simulink model "controller"  (R2016b)
settings: Solver=VariableStepAuto  StartTime=0.0  StopTime=10.0  RelTol=1e-3
undefined symbols (not defined in the file): D9, MaxSpeed, PTD5
libraries: simulink x7, frdmkl25zlib x2, slrtlib x2
settings Model: Creator=VasutornSIRIYAKORN  LastModifiedBy=VasutornSIRIYAKORN

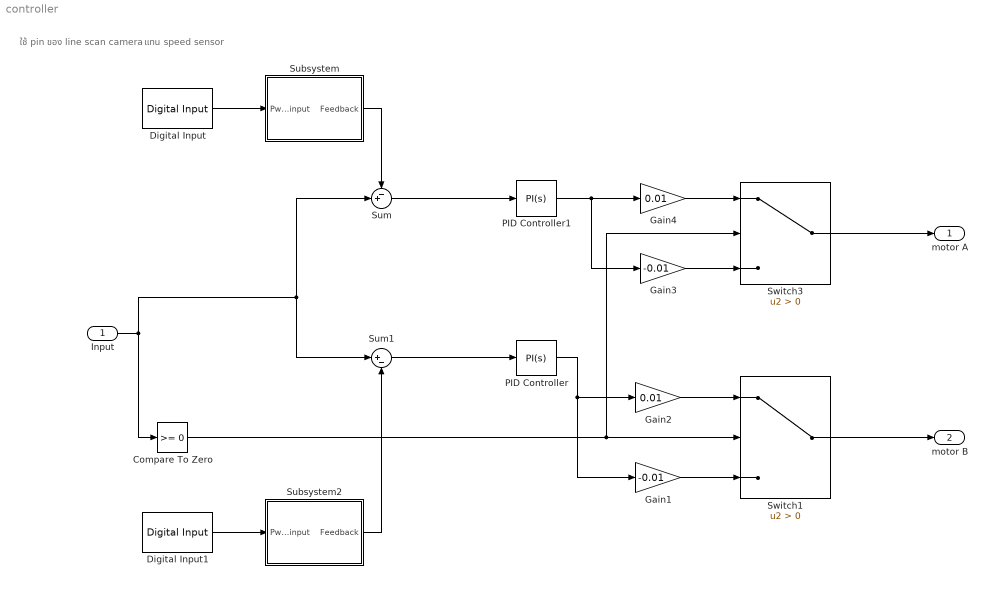
== system controller ==
  note: ใช้ pin ของ line scan camera แทน speed sensor
  "Input " : Inport
  Compare To Zero : simulink/Logic and Bit Operations/Compare To Zero  relop=>=  OutDataTypeStr=boolean
  Digital Input : frdmkl25zlib/Digital Input  Priority=2  WhichPin=PTD5 (D9)  SampleTime=0.01
  Digital Input1 : frdmkl25zlib/Digital Input  Priority=2  WhichPin=PTD7  SampleTime=0.01
  Gain1 : Gain  Gain=-0.01
  Gain2 : Gain  Gain=0.01
  Gain3 : Gain  Gain=-0.01
  Gain4 : Gain  Gain=0.01
  PID Controller : simulink/Continuous/PID Controller  Controller=PI  TimeDomain=Continuous-time  SampleTime=-1  IntegratorMethod=Forward Euler  FilterMethod=Forward Euler  Form=Parallel  UseFilter=on  ControllerParametersSource=internal  P=20  I=30  D=0  N=100  InitialConditionSource=internal  InitialConditionForIntegrator=0  InitialConditionForFilter=0  ExternalReset=none  LimitOutput=off  UpperSaturationLimit=inf  LowerSaturationLimit=-inf  LinearizeAsGain=on  AntiWindupMode=none  Kb=1  TrackingMode=off  Kt=1  PParamMin=[]  PParamMax=[]  IParamMin=[]  IParamMax=[]  DParamMin=[]  DParamMax=[]  NParamMin=[]  NParamMax=[]  KbParamMin=[]  KbParamMax=[]  KtParamMin=[]  KtParamMax=[]  POutMin=[]  POutMax=[]  IOutMin=[]  IOutMax=[]  DOutMin=[]  DOutMax=[]  NOutMin=[]  NOutMax=[]  KbOutMin=[]  KbOutMax=[]  KtOutMin=[]  KtOutMax=[]  IntegratorOutMin=[]  IntegratorOutMax=[]  FilterOutMin=[]  FilterOutMax=[]  SumOutMin=[]  SumOutMax=[]  SumI1OutMin=[]  SumI1OutMax=[]  SumI2OutMin=[]  SumI2OutMax=[]  SumI3OutMin=[]  SumI3OutMax=[]  SumDOutMin=[]  SumDOutMax=[]  SaturationOutMin=[]  SaturationOutMax=[]  IntegratorContinuousStateAttributes=''  IntegratorStateMustResolveToSignalObject=off  IntegratorRTWStateStorageClass=Auto  FilterContinuousStateAttributes=''  FilterStateMustResolveToSignalObject=off  FilterRTWStateStorageClass=Auto  DifferentiatorICPrevScaledInput=0  DifferentiatorOutMin=[]  DifferentiatorOutMax=[]
  PID Controller1 : simulink/Continuous/PID Controller  Controller=PI  TimeDomain=Continuous-time  SampleTime=-1  IntegratorMethod=Forward Euler  FilterMethod=Forward Euler  Form=Parallel  UseFilter=on  ControllerParametersSource=internal  P=20  I=30  D=0  N=100  InitialConditionSource=internal  InitialConditionForIntegrator=0  InitialConditionForFilter=0  ExternalReset=none  LimitOutput=off  UpperSaturationLimit=inf  LowerSaturationLimit=-inf  LinearizeAsGain=on  AntiWindupMode=none  Kb=1  TrackingMode=off  Kt=1  PParamMin=[]  PParamMax=[]  IParamMin=[]  IParamMax=[]  DParamMin=[]  DParamMax=[]  NParamMin=[]  NParamMax=[]  KbParamMin=[]  KbParamMax=[]  KtParamMin=[]  KtParamMax=[]  POutMin=[]  POutMax=[]  IOutMin=[]  IOutMax=[]  DOutMin=[]  DOutMax=[]  NOutMin=[]  NOutMax=[]  KbOutMin=[]  KbOutMax=[]  KtOutMin=[]  KtOutMax=[]  IntegratorOutMin=[]  IntegratorOutMax=[]  FilterOutMin=[]  FilterOutMax=[]  SumOutMin=[]  SumOutMax=[]  SumI1OutMin=[]  SumI1OutMax=[]  SumI2OutMin=[]  SumI2OutMax=[]  SumI3OutMin=[]  SumI3OutMax=[]  SumDOutMin=[]  SumDOutMax=[]  SaturationOutMin=[]  SaturationOutMax=[]  IntegratorContinuousStateAttributes=''  IntegratorStateMustResolveToSignalObject=off  IntegratorRTWStateStorageClass=Auto  FilterContinuousStateAttributes=''  FilterStateMustResolveToSignalObject=off  FilterRTWStateStorageClass=Auto  DifferentiatorICPrevScaledInput=0  DifferentiatorOutMin=[]  DifferentiatorOutMax=[]
  Subsystem : Subsystem
  Subsystem2 : Subsystem
  Sum : Sum  Inputs=-+|
  Sum1 : Sum  Inputs=|+-
  Switch1 : Switch  Criteria=u2 > Threshold
  Switch3 : Switch  Criteria=u2 > Threshold
  motor A : Outport
  "motor B " : Outport  Port=2
  wires:
  Subsystem/1(Feedback) -> Sum/1
  Digital Input/1 -> Subsystem/1(Pwm input)
  Sum/1 -> PID Controller1/1
  "Input "/1 -> Sum1/1, Sum/2, Compare To Zero/1
  Digital Input1/1 -> Subsystem2/1(Pwm input)
  Sum1/1 -> PID Controller/1
  Subsystem2/1(Feedback) -> Sum1/2
  Gain2/1 -> Switch1/1
  Gain1/1 -> Switch1/3
  Switch1/1 -> "motor B "/1
  PID Controller1/1 -> Gain4/1, Gain3/1
  PID Controller/1 -> Gain1/1, Gain2/1
  Gain4/1 -> Switch3/1
  Gain3/1 -> Switch3/3
  Switch3/1 -> motor A/1
  Compare To Zero/1 -> Switch3/2, Switch1/2

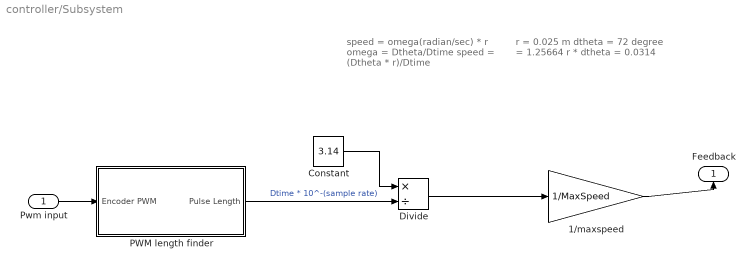
== system controller/Subsystem ==
  note: r = 0.025 m
      | dtheta = 72 degree = 1.25664
      | r * dtheta = 0.0314
  note: speed = omega(radian/sec) * r
      | omega = Dtheta/Dtime
      | speed = (Dtheta * r)/Dtime
  Pwm input : Inport
  1/maxspeed : Gain  Gain=1/MaxSpeed
  Constant : Constant  Value=3.14
  Divide : Product  Inputs=*/
  PWM length finder : Subsystem
  Feedback : Outport
  wires:
  Pwm input/1 -> PWM length finder/1(Encoder PWM)
  Divide/1 -> 1/maxspeed/1
  Constant/1 -> Divide/1
  PWM length finder/1(Pulse Length) -> Divide/2  "Dtime * 10^-(sample rate)"
  1/maxspeed/1 -> Feedback/1

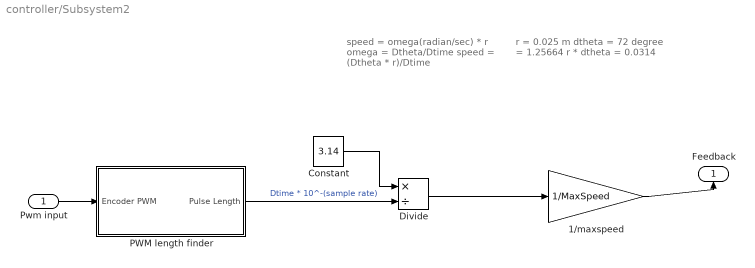
== system controller/Subsystem2 ==
  note: r = 0.025 m
      | dtheta = 72 degree = 1.25664
      | r * dtheta = 0.0314
  note: speed = omega(radian/sec) * r
      | omega = Dtheta/Dtime
      | speed = (Dtheta * r)/Dtime
  Pwm input : Inport
  1/maxspeed : Gain  Gain=1/MaxSpeed
  Constant : Constant  Value=3.14
  Divide : Product  Inputs=*/
  PWM length finder : Subsystem
  Feedback : Outport
  wires:
  Pwm input/1 -> PWM length finder/1(Encoder PWM)
  Divide/1 -> 1/maxspeed/1
  Constant/1 -> Divide/1
  PWM length finder/1(Pulse Length) -> Divide/2  "Dtime * 10^-(sample rate)"
  1/maxspeed/1 -> Feedback/1

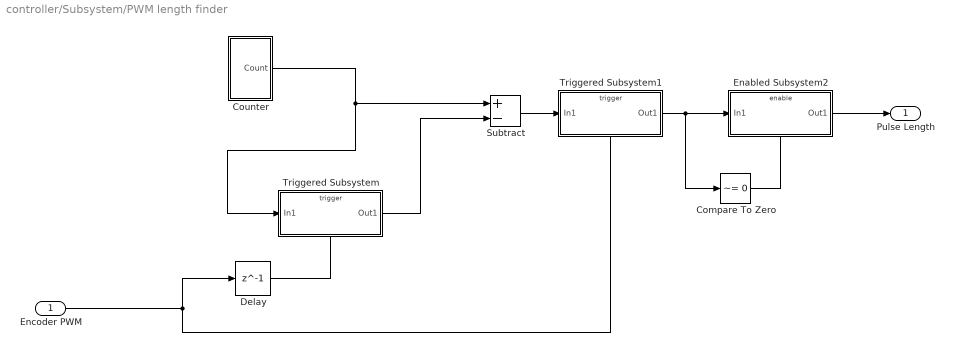
== system controller/Subsystem/PWM length finder ==
  Encoder PWM : Inport
  Compare To Zero : simulink/Logic and Bit Operations/Compare To Zero  relop=~=  OutDataTypeStr=boolean
  "Counter " : Subsystem
  Delay : Delay  DelayLength=1  InitialCondition=0  SampleTime=0.01
  Enabled Subsystem2 : Subsystem  TreatAsAtomicUnit=on
  Subtract : Sum  Inputs=+-
  Triggered Subsystem : Subsystem  TreatAsAtomicUnit=on
  Triggered Subsystem1 : Subsystem  TreatAsAtomicUnit=on
  Pulse Length : Outport
  wires:
  Delay/1 -> Triggered Subsystem/Trigger
  Encoder PWM/1 -> Delay/1, Triggered Subsystem1/Trigger
  Compare To Zero/1 -> Enabled Subsystem2/Enable
  Enabled Subsystem2/1(Out1) -> Pulse Length/1
  Triggered Subsystem1/1(Out1) -> Compare To Zero/1, Enabled Subsystem2/1(In1)
  Triggered Subsystem/1(Out1) -> Subtract/2
  "Counter "/1(Count) -> Subtract/1, Triggered Subsystem/1(In1)
  Subtract/1 -> Triggered Subsystem1/1(In1)

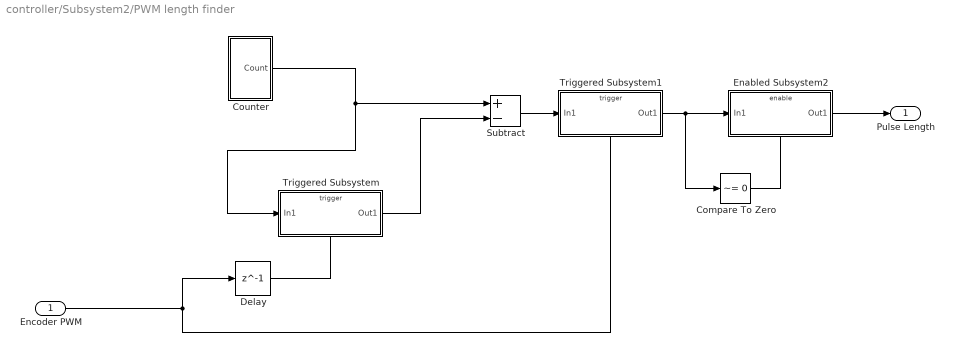
== system controller/Subsystem2/PWM length finder ==
  Encoder PWM : Inport
  Compare To Zero : simulink/Logic and Bit Operations/Compare To Zero  relop=~=  OutDataTypeStr=boolean
  "Counter " : Subsystem
  Delay : Delay  DelayLength=1  InitialCondition=0  SampleTime=0.01
  Enabled Subsystem2 : Subsystem  TreatAsAtomicUnit=on
  Subtract : Sum  Inputs=+-
  Triggered Subsystem : Subsystem  TreatAsAtomicUnit=on
  Triggered Subsystem1 : Subsystem  TreatAsAtomicUnit=on
  Pulse Length : Outport
  wires:
  Delay/1 -> Triggered Subsystem/Trigger
  Encoder PWM/1 -> Delay/1, Triggered Subsystem1/Trigger
  Compare To Zero/1 -> Enabled Subsystem2/Enable
  Enabled Subsystem2/1(Out1) -> Pulse Length/1
  Triggered Subsystem1/1(Out1) -> Compare To Zero/1, Enabled Subsystem2/1(In1)
  Triggered Subsystem/1(Out1) -> Subtract/2
  "Counter "/1(Count) -> Subtract/1, Triggered Subsystem/1(In1)
  Subtract/1 -> Triggered Subsystem1/1(In1)

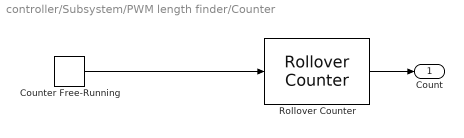
== system controller/Subsystem/PWM length finder/Counter  ==
  Counter Free-Running : simulink/Sources/Counter Free-Running  NumBits=16  tsamp=0.01
  "Rollover Counter " : slrtlib/Incremental Encoder/Utilities/Rollover/Rollover Counter   InitialValue=0  RolloverThreshold=2^15
  Count : Outport
  wires:
  Counter Free-Running/1 -> "Rollover Counter "/1
  "Rollover Counter "/1 -> Count/1

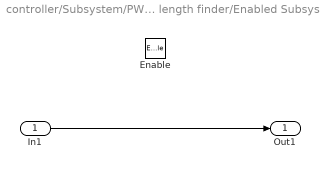
== system controller/Subsystem/PWM length finder/Enabled Subsystem2 ==
  In1 : Inport
  Enable : EnablePort
  Out1 : Outport
  wires:
  In1/1 -> Out1/1

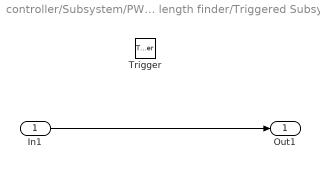
== system controller/Subsystem/PWM length finder/Triggered Subsystem ==
  In1 : Inport
  Trigger : TriggerPort  TriggerType=falling  VariantControl=Variant
  Out1 : Outport
  wires:
  In1/1 -> Out1/1

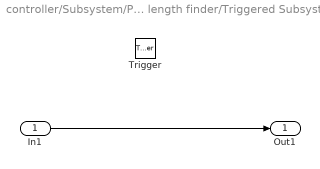
== system controller/Subsystem/PWM length finder/Triggered Subsystem1 ==
  In1 : Inport
  Trigger : TriggerPort  TriggerType=falling  VariantControl=Variant
  Out1 : Outport
  wires:
  In1/1 -> Out1/1

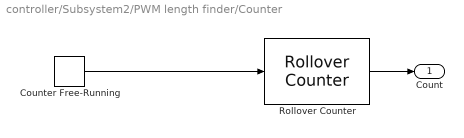
== system controller/Subsystem2/PWM length finder/Counter  ==
  Counter Free-Running : simulink/Sources/Counter Free-Running  NumBits=16  tsamp=0.01
  "Rollover Counter " : slrtlib/Incremental Encoder/Utilities/Rollover/Rollover Counter   InitialValue=0  RolloverThreshold=2^15
  Count : Outport
  wires:
  Counter Free-Running/1 -> "Rollover Counter "/1
  "Rollover Counter "/1 -> Count/1

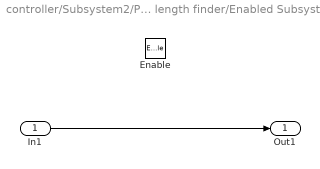
== system controller/Subsystem2/PWM length finder/Enabled Subsystem2 ==
  In1 : Inport
  Enable : EnablePort
  Out1 : Outport
  wires:
  In1/1 -> Out1/1

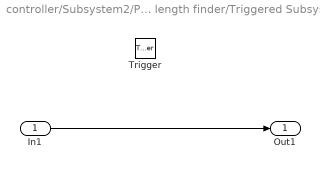
== system controller/Subsystem2/PWM length finder/Triggered Subsystem ==
  In1 : Inport
  Trigger : TriggerPort  TriggerType=falling  VariantControl=Variant
  Out1 : Outport
  wires:
  In1/1 -> Out1/1

== system controller/Subsystem2/PWM length finder/Triggered Subsystem1 ==
  In1 : Inport
  Trigger : TriggerPort  TriggerType=falling  VariantControl=Variant
  Out1 : Outport
  wires:
  In1/1 -> Out1/1
